simulink model "phys0712"  (R2024a)
settings: Solver=VariableStepAuto  StartTime=0.0  StopTime=150  RelTol=1e-3
settings Model: Creator=pupkinzalupkin  LastModifiedBy=pupkinzalupkin

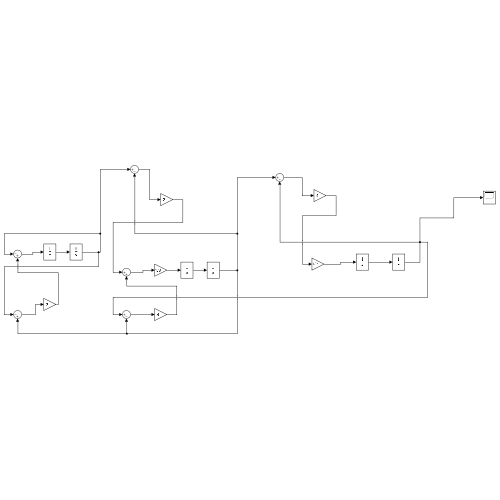
[thumbnail: Simulink's stored preview of the top-level diagram]
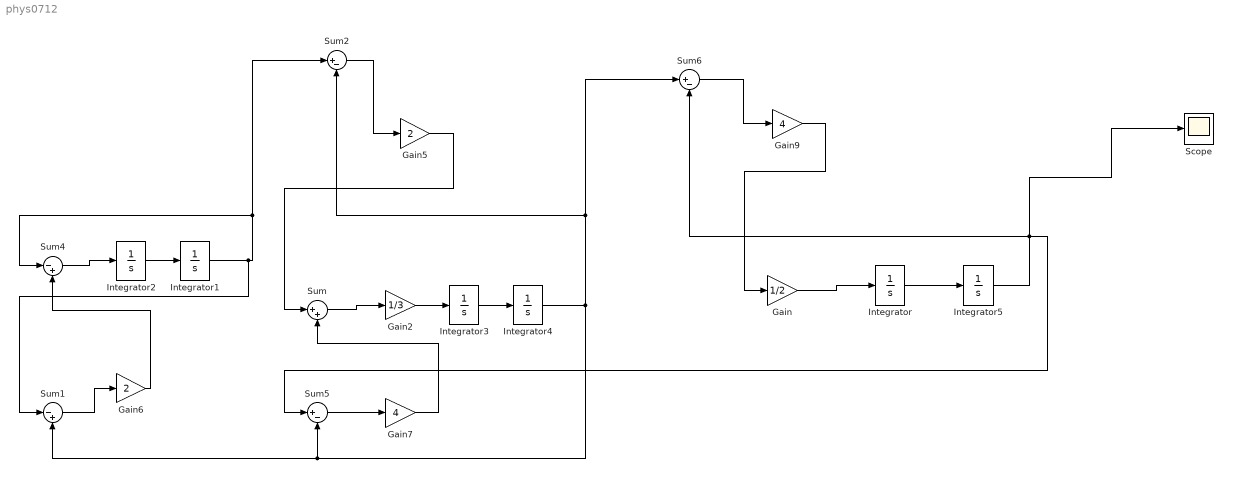
== system phys0712 ==
  Gain : Gain  Gain=1/2
  Gain2 : Gain  Gain=1/3
  Gain5 : Gain  Gain=2
  Gain6 : Gain  Gain=2
  Gain7 : Gain  Gain=4
  Gain9 : Gain  Gain=4
  Integrator{,2..5} (5 alike) : Integrator
  Integrator1 : Integrator  InitialCondition=1
  Scope : Scope
  Sum : Sum  Inputs=|++
  Sum1 : Sum  Inputs=|-+
  Sum2 : Sum  Inputs=|+-
  Sum4 : Sum  Inputs=|-+
  Sum5 : Sum  Inputs=|+-
  Sum6 : Sum  Inputs=|+-
  wires:
  Gain/1 -> Integrator/1
  Sum/1 -> Gain2/1
  Gain2/1 -> Integrator3/1
  Integrator5/1 -> Sum5/1, Scope/1, Sum6/2
  Sum1/1 -> Gain6/1
  Gain6/1 -> Sum4/2
  Sum4/1 -> Integrator2/1
  Sum2/1 -> Gain5/1
  Gain5/1 -> Sum/1
  Sum5/1 -> Gain7/1
  Gain7/1 -> Sum/2
  Sum6/1 -> Gain9/1
  Integrator2/1 -> Integrator1/1
  Integrator3/1 -> Integrator4/1
  Integrator/1 -> Integrator5/1
  Gain9/1 -> Gain/1
  Integrator1/1 -> Sum1/1, Sum4/1, Sum2/1
  Integrator4/1 -> Sum5/2, Sum1/2, Sum2/2, Sum6/1
